simulink model "quad_12_1_r2021a"  (R2022a)
settings: Solver=ode4  StartTime=0.0  StopTime=120  FixedStep=0.001  RelTol=1e-3
values from neighbouring files (symbols this model uses):
  Ixc = 9373.661914436/1e6    (= 0.00937366191444)    [ParamsInit_test.m]
  Iyc = 11755.067703159/1e6    (= 0.0117550677032)    [ParamsInit_test.m]
  Izc = 17533.553367555/1e6    (= 0.0175335533676)    [ParamsInit_test.m]
  kd_h = damp_ratio_h*2*sqrt(kp_h*Vehicle.Airframe.mass)    [ParamsInit_test.m]
  kd_phi = damp_ratio_phi*2*sqrt(kp_phi*Ixc)    [ParamsInit_test.m]
  kd_theta = damp_ratio_theta*2*sqrt(kp_theta*Iyc)    [ParamsInit_test.m]
  kd_yaw = damp_ratio_yaw*2*sqrt(kp_yaw*Izc)    [ParamsInit_test.m]
  kp_h = omega_n_h^2*Vehicle.Airframe.mass    [ParamsInit_test.m]
  kp_phi = omega_n_phi^2*Ixc    (= 0.937366191444)    [ParamsInit_test.m]
  kp_position = 0.1    [ParamsInit_test.m]
  kp_theta = omega_n_theta^2*Iyc    (= 1.17550677032)    [ParamsInit_test.m]
  kp_vx = 0.25    [ParamsInit_test.m]
  kp_vy = 0.25    [ParamsInit_test.m]
  kp_yaw = omega_n_yaw^2*Izc    (= 0.0175335533676)    [ParamsInit_test.m]
undefined symbols (not defined in the file or in its folder): Vehicle
libraries: simulink x3, aerolibnav x3, aerolibconvert2 x2, mspfiltlib x1, sensorgpslib x1, mspsensorlib x1, sensorinslib x1, aerolibasang x1, sharedtransform x1, aerolibanimutils x1, uavutilslib x1
settings Model: Creator=gaowe  LastModifiedBy=GMS
settings SolverCC: AlgebraicLoopSolver=TrustRegion
settings RTWCC: DLArmComputeVersion=19.05

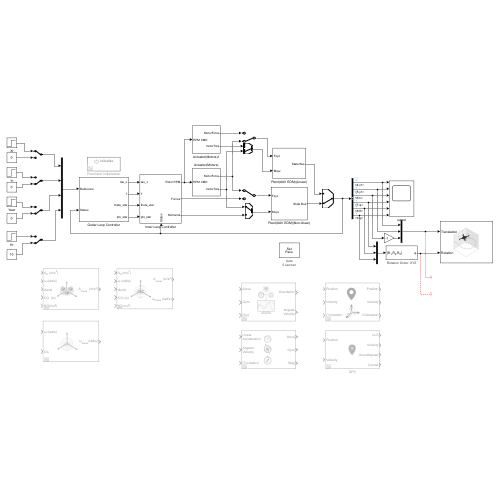
[thumbnail: Simulink's stored preview of the top-level diagram]
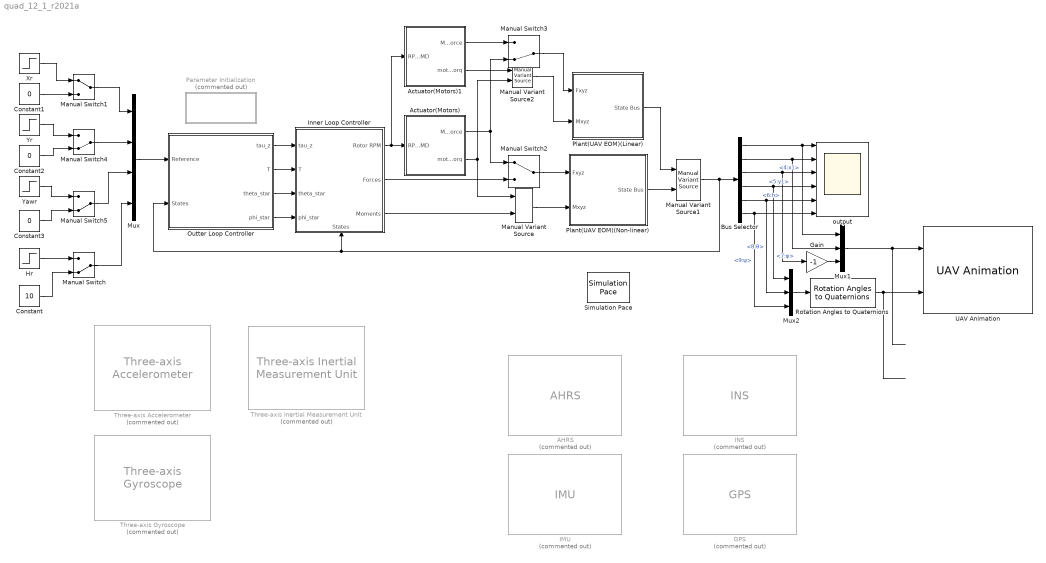
== system quad_12_1_r2021a ==
  AHRS : mspfiltlib/AHRS  Commented=on  DispRefFrame=NED  DecimationFactor=1  InitialProcessNoise=ahrsfilter.defaultProcessNoise  OrientationFormat=quaternion  SimulateUsing=Interpreted execution  AccelerometerNoise=0.0001924722  GyroscopeNoise=9.1385e-5  MagnetometerNoise=0.1  GyroscopeDriftNoise=3.0462e-13  LinearAccelerationNoise=0.0096236100000000012  MagneticDisturbanceNoise=0.5  LinearAccelerationDecayFactor=0.5  MagneticDisturbanceDecayFactor=0.5  ExpectedMagneticFieldStrength=50
  Actuator(Motors) : Subsystem
  Actuator(Motors)1 : Subsystem
  Bus Selector : BusSelector  OutputSignals=4:x1,5:y1,6:h,7:φ,8:θ,9:ψ
  Constant : Constant  Value=10
  Constant1 : Constant  Value=0
  Constant2 : Constant  Value=0
  Constant3 : Constant  Value=0
  GPS : sensorgpslib/GPS  Commented=on  DispRefFrame=NED  PositionInputFormat=Local  ReferenceLocation=[ 0, 0, 0 ]  HorizontalPositionAccuracy=1.6  VerticalPositionAccuracy=3  VelocityAccuracy=0.1  DecayFactor=0.999  SeedDouble=67  SimulateUsing=Interpreted execution
  Gain : Gain  Gain=-1
  Hr : Step  Time=0  After=20  SampleTime=0
  IMU : mspsensorlib/IMU  Commented=on  DispRefFrame=NED  Temperature=25  MagneticFieldNED=[ 27.5550, -2.4169, -16.0849 ]  MagneticFieldENU=[ -2.4169, 27.5550, 16.0849 ]  SeedDouble=67  SimulateUsing=Interpreted execution  AccelParamsMeasurementRange=Inf  AccelParamsResolution=0  AccelParamsConstantBias=[ 0, 0, 0 ]  AccelParamsAxesMisalignment=[ 100, 0, 0; 0, 100, 0; 0, 0, 100 ]  AccelParamsNoiseDensity=[ 0, 0, 0 ]  AccelParamsBiasInstability=[ 0, 0, 0 ]  AccelParamsRandomWalk=[ 0, 0, 0 ]  AccelParamsTemperatureBias=[ 0, 0, 0 ]  AccelParamsTemperatureScaleFactor=[ 0, 0, 0 ]  GyroParamsMeasurementRange=Inf  GyroParamsResolution=0  GyroParamsConstantBias=[ 0, 0, 0 ]  GyroParamsAxesMisalignment=[ 100, 0, 0; 0, 100, 0; 0, 0, 100 ]  GyroParamsAccelerationBias=[ 0, 0, 0 ]  GyroParamsNoiseDensity=[ 0, 0, 0 ]  GyroParamsBiasInstability=[ 0, 0, 0 ]  GyroParamsRandomWalk=[ 0, 0, 0 ]  GyroParamsTemperatureBias=[ 0, 0, 0 ]  GyroParamsTemperatureScaleFactor=[ 0, 0, 0 ]  MagParamsMeasurementRange=Inf  MagParamsResolution=0  MagParamsConstantBias=[ 0, 0, 0 ]  MagParamsAxesMisalignment=[ 100, 0, 0; 0, 100, 0; 0, 0, 100 ]  MagParamsNoiseDensity=[ 0, 0, 0 ]  MagParamsBiasInstability=[ 0, 0, 0 ]  MagParamsRandomWalk=[ 0, 0, 0 ]  MagParamsTemperatureBias=[ 0, 0, 0 ]  MagParamsTemperatureScaleFactor=[ 0, 0, 0 ]
  INS : sensorinslib/INS  Commented=on  MountingLocation=[0 0 0]  RollAccuracy=0.2  PitchAccuracy=0.2  YawAccuracy=1  PositionAccuracy=1  VelocityAccuracy=0.05  UseAccelAndAngVel=off  AccelerationAccuracy=0  AngularVelocityAccuracy=0  TimeInput=off  PositionErrorFactor=[0 0 0]  SeedDouble=67  SimulateUsing=Interpreted execution
  Inner Loop Controller : Subsystem
      settings: PortSchema="{\"entries\":[{\"content\":{\"sides\":[{\"content\":{\"connectorIds\":[\"In1\",\"In2\",\"In3\",\"In4\"]},\"type\":\"ConnectorPlacement.EquallySpacedRectSide\",\"uuid\":\"3024e14a-e42b-4ece-95b6-8188e577f7ea\"},{\"content\":{\"connectorIds\":[\"Out1\",\"Out2\",\"Out3\"],\"side\":\"RIGHT\"},\"type\":\"ConnectorPlacement.EquallySpacedRectSide\",\"uuid\":\"28791f10-00d9-435c-9b3a-62150bd300bc\"},{\"content\":{\"connectorIds\":[],\"side\":\"TOP\"},\"type\":\"ConnectorPlacement.EquallySpacedRectSide\",\"uuid\":\"5a81466d-668a-47df-a46c-2854fa138474\"},{\"content\":{\"connectorIds\":[\"In5\"],\"side\":\"BOTTOM\"},\"type\":\"ConnectorPlacement.EquallySpacedRectSide\",\"uuid\":\"dc01fcce-ea7b-43d7-98f8-2115160ba315\"}]},\"type\":\"ConnectorPlacement.EquallySpacedConnector\",\"uuid\":\"802a1a82-5ed7-4d3a-8fbf-5749d0aa0952\"}],\"packageUris\":[\"http://schema.mathworks.com/mf0/Connector/R2020b\"],\"version\":\"1.0\"}"
  Manual Variant Source : simulink/Signal Routing/Manual Variant Source  NumChoices=2  LabelModeActiveChoice=V_1
  Manual Variant Source1 : simulink/Signal Routing/Manual Variant Source  NumChoices=2  LabelModeActiveChoice=V_2
  Manual Variant Source2 : simulink/Signal Routing/Manual Variant Source  NumChoices=2  LabelModeActiveChoice=V_2
  Manual Switch{,3..5} (4 alike) : ManualSwitch  CurrentSetting=0
  Manual Switch1 : ManualSwitch
  Manual Switch2 : ManualSwitch
  Mux : Mux
  Mux1 : Mux  Inputs=3
  Mux2 : Mux  Inputs=3
  Outter Loop Controller : Subsystem
  Parameter Initialization : Subsystem  Commented=on  TreatAsAtomicUnit=on
  Plant(UAV EOM)(Linear) : Subsystem
  Plant(UAV EOM)(Non-linear) : Subsystem
  Rotation Angles to Quaternions : sharedtransform/Rotation Angles to Quaternions  rotationOrder=XYZ  aMode=aMode
  Simulation Pace : aerolibanimutils/Simulation Pace  SimulationPace=5  SleepMode=Auto  OutputPaceError=off  SampleTime=1/100
  Three-axis Accelerometer : aerolibnav/Three-axis Accelerometer  Commented=on  units=Metric (MKS)  acc=[0 0 0]  gtype=on  dtype_a=on  w_a=190  z_a=0.707  a_sf_cc=[1 0 0; 0 1 0; 0 0 1]  a_bias=[0 0 0]  a_Ts=0  a_rand=on  a_seeds=[23093 23094 23095]  a_pow=[0.001 0.001 0.001]  a_sat="[-inf  -inf  -inf  inf inf inf]"
  Three-axis Gyroscope : aerolibnav/Three-axis Gyroscope  Commented=on  dtype_g=on  w_g=190  z_g=0.707  g_sf_cc=[1 0 0; 0 1 0; 0 0 1]  g_bias=[0 0 0]  g_sen=[0 0 0]  g_Ts=0  g_rand=on  g_seeds=[23093 23094 23095]  g_pow=[0.0001 0.0001 0.0001]  g_sat="[-inf  -inf  -inf  inf inf inf]"
  Three-axis Inertial Measurement Unit : aerolibnav/Three-axis Inertial Measurement Unit  Commented=on  units=Metric (MKS)  imu=[0 0 0]  i_Ts=0  dtype_a=on  w_a=190  z_a=0.707  a_sf_cc=[1 0 0; 0 1 0; 0 0 1]  a_bias=[0 0 0]  a_sat="[-inf  -inf  -inf  inf inf inf]"  dtype_g=on  w_g=190  z_g=0.707  g_sf_cc=[1 0 0; 0 1 0; 0 0 1]  g_bias=[0 0 0]  g_sens=[0 0 0]  g_sat="[-inf  -inf  -inf  inf inf inf]"  i_rand=on  i_seeds=[23093 23094 23095 23096 23097 23098]  i_pow=[0.001 0.001 0.001 0.0001 0.0001 0.0001]
  UAV Animation : uavutilslib/UAV Animation  UAVType=Multirotor  UAVSize=1  InertialZDirection=Down  SampleTime=1/100
  Xr : Step  Time=0  After=10  SampleTime=0
  Yawr : Step  Time=0  After=pi/2  SampleTime=0
  Yr : Step  Time=0  After=10  SampleTime=0
  output : Scope  NumInputPorts=6
  wires:
  Manual Variant Source1/1 -> Outter Loop Controller/2(States), Inner Loop Controller/5(States), Bus Selector/1
  Mux/1 -> Outter Loop Controller/1(Reference)
  Manual Switch1/1 -> Mux/1
  Constant2/1 -> Manual Switch4/2
  Yawr/1 -> Manual Switch5/1
  Hr/1 -> Manual Switch/1
  Outter Loop Controller/3(theta_star) -> Inner Loop Controller/3(theta_star)
  Outter Loop Controller/1(tau_z) -> Inner Loop Controller/1(tau_z)
  Outter Loop Controller/2(T) -> Inner Loop Controller/2(T)
  Outter Loop Controller/4(phi_star) -> Inner Loop Controller/4(phi_star)
  Inner Loop Controller/1(Rotor RPM) -> Actuator(Motors)1/1(RPM CMD), Actuator(Motors)/1(RPM CMD)
  Actuator(Motors)/1(MotorForce) -> Manual Switch3/2, Manual Switch2/1
  Actuator(Motors)/2(motorTorq) -> Manual Variant Source2/2, Manual Variant Source/1
  Bus Selector/1 -> Mux1/1, output/1  "<4:x1>"
  Bus Selector/2 -> Mux1/2, output/2  "<5:y1>"
  Bus Selector/3 -> Gain/1, output/3  "<6:h>"
  Bus Selector/4 -> Mux2/1, output/4  "<7:φ>"
  Bus Selector/5 -> Mux2/2, output/5  "<8:θ>"
  Bus Selector/6 -> Mux2/3, output/6  "<9:ψ>"
  Manual Switch/1 -> Mux/4
  Constant/1 -> Manual Switch/2
  Constant1/1 -> Manual Switch1/2
  Xr/1 -> Manual Switch1/1
  Inner Loop Controller/2(Forces) -> Manual Switch2/2
  Inner Loop Controller/3(Moments) -> Manual Variant Source/2
  Plant(UAV EOM)(Linear)/1(State Bus) -> Manual Variant Source1/1
  Manual Variant Source/1 -> Plant(UAV EOM)(Non-linear)/2(Mxyz)
  Manual Switch2/1 -> Plant(UAV EOM)(Non-linear)/1(Fxyz)
  Plant(UAV EOM)(Non-linear)/1(State Bus) -> Manual Variant Source1/2
  Actuator(Motors)1/1(MotorForce) -> Manual Switch3/1
  Actuator(Motors)1/2(motorTorq) -> Manual Variant Source2/1
  Manual Switch3/1 -> Plant(UAV EOM)(Linear)/1(Fxyz)
  Manual Variant Source2/1 -> Plant(UAV EOM)(Linear)/2(Mxyz)
  Manual Switch4/1 -> Mux/2
  Yr/1 -> Manual Switch4/1
  Constant3/1 -> Manual Switch5/2
  Manual Switch5/1 -> Mux/3
  Mux1/1 -> UAV Animation/1
  Rotation Angles to Quaternions/1 -> UAV Animation/2
  Mux2/1 -> Rotation Angles to Quaternions/1
  Gain/1 -> Mux1/3

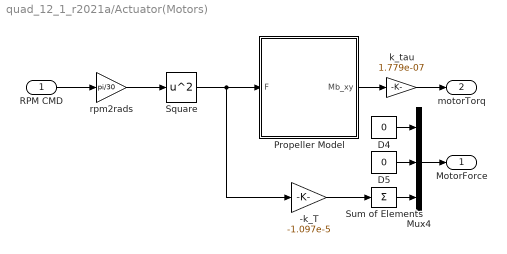
== system quad_12_1_r2021a/Actuator(Motors) ==
  RPM CMD : Inport
  -k_T : Gain  Gain=-1.097e-5
  D4 : Constant  Value=0
  D5 : Constant  Value=0
  Mux4 : Mux  Inputs=3
  Propeller Model : MATLAB Function  TreatAsAtomicUnit=on
  Square : Math  Operator=square
  Sum of Elements : Sum  Inputs=+
  k_tau : Gain  Gain=1.779e-07
  rpm2rads : Gain  Gain=pi/30
  MotorForce : Outport
  motorTorq : Outport  Port=2
  wires:
  k_tau/1 -> motorTorq/1
  Mux4/1 -> MotorForce/1
  Sum of Elements/1 -> Mux4/3
  -k_T/1 -> Sum of Elements/1
  Square/1 -> -k_T/1, Propeller Model/1(F)
  Propeller Model/1(Mb_xy) -> k_tau/1
  D4/1 -> Mux4/1
  D5/1 -> Mux4/2
  RPM CMD/1 -> rpm2rads/1
  rpm2rads/1 -> Square/1

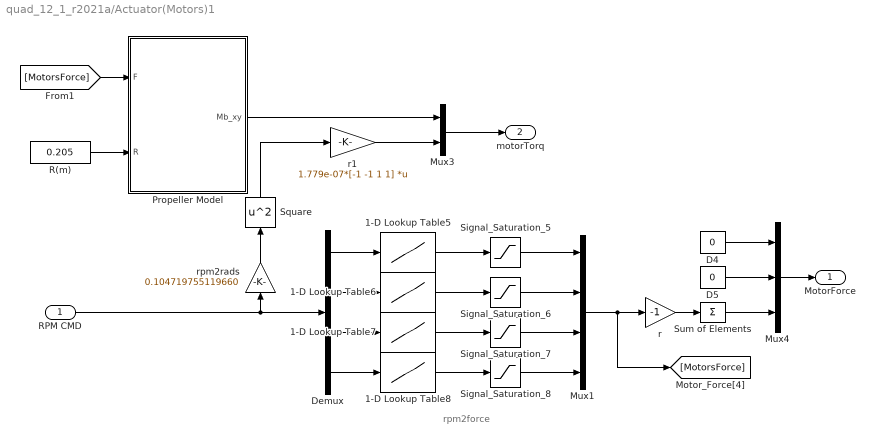
== system quad_12_1_r2021a/Actuator(Motors)1 ==
  note: rpm2force
  RPM CMD : Inport
  1-D Lookup Table5 : Lookup_n-D  NumberOfTableDimensions=1  BreakpointsForDimension1=|  BeginIndexSearchUsingPreviousIndexResult=on  Table=|  InternalRulePriority=Speed  RndMeth=Simplest
      BreakpointsForDimension1=|
      | [2847
      | 3689
      | 4585
      | 5400
      | 6400
      | 7000
      | 7800
      | 8222
      | 9300
      | 10700]
      Table=|
      | [0.6664
      | 1.4308
      | 2.3422
      | 3.3418
      | 4.9098
      | 5.929
      | 7.399
      | 7.6244
      | 10.976
      | 13.72]
  1-D Lookup Table6 : Lookup_n-D  NumberOfTableDimensions=1  BreakpointsForDimension1=|  BeginIndexSearchUsingPreviousIndexResult=on  Table=|  InternalRulePriority=Speed  RndMeth=Simplest
      BreakpointsForDimension1=|
      | [2847
      | 3689
      | 4585
      | 5400
      | 6400
      | 7000
      | 7800
      | 8222
      | 9300
      | 10700]
      Table=|
      | [0.6664
      | 1.4308
      | 2.3422
      | 3.3418
      | 4.9098
      | 5.929
      | 7.399
      | 7.6244
      | 10.976
      | 13.72]
  1-D Lookup Table7 : Lookup_n-D  NumberOfTableDimensions=1  BreakpointsForDimension1=|  BeginIndexSearchUsingPreviousIndexResult=on  Table=|  InternalRulePriority=Speed  RndMeth=Simplest
      BreakpointsForDimension1=|
      | [2847
      | 3689
      | 4585
      | 5400
      | 6400
      | 7000
      | 7800
      | 8222
      | 9300
      | 10700]
      Table=|
      | [0.6664
      | 1.4308
      | 2.3422
      | 3.3418
      | 4.9098
      | 5.929
      | 7.399
      | 7.6244
      | 10.976
      | 13.72]
  1-D Lookup Table8 : Lookup_n-D  NumberOfTableDimensions=1  BreakpointsForDimension1=|  BeginIndexSearchUsingPreviousIndexResult=on  Table=|  InternalRulePriority=Speed  RndMeth=Simplest
      BreakpointsForDimension1=|
      | [2847
      | 3689
      | 4585
      | 5400
      | 6400
      | 7000
      | 7800
      | 8222
      | 9300
      | 10700]
      Table=|
      | [0.6664
      | 1.4308
      | 2.3422
      | 3.3418
      | 4.9098
      | 5.929
      | 7.399
      | 7.6244
      | 10.976
      | 13.72]
  D4 : Constant  Value=0
  D5 : Constant  Value=0
  Demux : Demux
  Mux1 : Mux
  Mux3 : Mux  Inputs=[2 1]
  Mux4 : Mux  Inputs=3
  Propeller Model : MATLAB Function  TreatAsAtomicUnit=on
  R(m) : Constant  Value=0.205
  Signal_Saturation_{5..8} (4 alike) : Saturate  UpperLimit=1.4*9.8  LowerLimit=0
  Square : Math  Operator=square
  Sum of Elements : Sum  Inputs=+
  r : Gain  Gain=-1
  r1 : Gain  Gain=1.779e-07*[-1 -1 1 1]  Multiplication=Matrix(K*u)
  rpm2rads : Gain  Gain=0.104719755119660
  MotorForce : Outport
  motorTorq : Outport  Port=2
  wires:
  Signal_Saturation_6/1 -> Mux1/2
  1-D Lookup Table7/1 -> Signal_Saturation_7/1
  Mux3/1 -> motorTorq/1
  1-D Lookup Table6/1 -> Signal_Saturation_6/1
  Mux4/1 -> MotorForce/1
  r1/1 -> Mux3/2
  Sum of Elements/1 -> Mux4/3
  r/1 -> Sum of Elements/1
  Mux1/1 -> [MotorsForce], r/1
  Demux/1 -> 1-D Lookup Table5/1
  Square/1 -> r1/1
  1-D Lookup Table5/1 -> Signal_Saturation_5/1
  Demux/3 -> 1-D Lookup Table7/1
  Signal_Saturation_5/1 -> Mux1/1
  1-D Lookup Table8/1 -> Signal_Saturation_8/1
  [MotorsForce] -> Propeller Model/1(F)
  Demux/4 -> 1-D Lookup Table8/1
  Demux/2 -> 1-D Lookup Table6/1
  Signal_Saturation_7/1 -> Mux1/3
  Propeller Model/1(Mb_xy) -> Mux3/1
  Signal_Saturation_8/1 -> Mux1/4
  R(m)/1 -> Propeller Model/2(R)
  D4/1 -> Mux4/1
  D5/1 -> Mux4/2
  RPM CMD/1 -> Demux/1, rpm2rads/1
  rpm2rads/1 -> Square/1

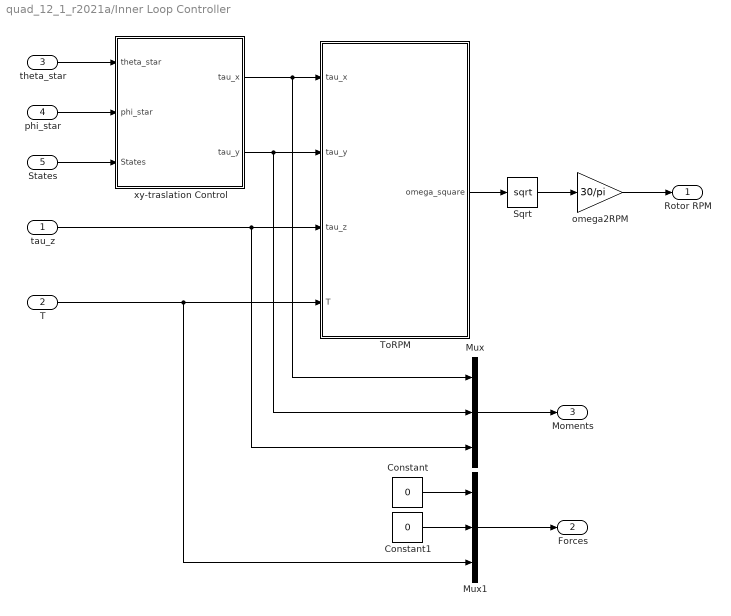
== system quad_12_1_r2021a/Inner Loop Controller ==
  tau_z : Inport
  T : Inport  Port=2
  theta_star : Inport  Port=3
  phi_star : Inport  Port=4
  States : Inport  Port=5
  Constant : Constant  Value=0
  Constant1 : Constant  Value=0
  Mux : Mux  Inputs=3
  Mux1 : Mux  Inputs=3
  Sqrt : Sqrt
  ToRPM : MATLAB Function  TreatAsAtomicUnit=on
  omega2RPM : Gain  Gain=30/pi
  xy-traslation Control : Subsystem
  Rotor RPM : Outport
  Forces : Outport  Port=2
  Moments : Outport  Port=3
  wires:
  theta_star/1 -> xy-traslation Control/1(theta_star)
  States/1 -> xy-traslation Control/3(States)
  phi_star/1 -> xy-traslation Control/2(phi_star)
  tau_z/1 -> Mux/3, ToRPM/3(tau_z)
  xy-traslation Control/2(tau_y) -> Mux/2, ToRPM/2(tau_y)
  xy-traslation Control/1(tau_x) -> Mux/1, ToRPM/1(tau_x)
  Sqrt/1 -> omega2RPM/1
  omega2RPM/1 -> Rotor RPM/1
  ToRPM/1(omega_square) -> Sqrt/1
  Mux/1 -> Moments/1
  Constant/1 -> Mux1/1
  Constant1/1 -> Mux1/2
  Mux1/1 -> Forces/1
  T/1 -> Mux1/3, ToRPM/4(T)

== system quad_12_1_r2021a/Outter Loop Controller ==
  Reference : Inport
  States : Inport  Port=2
  Demux : Demux
  Height Control : Subsystem
  Position Control : Subsystem
  Velocity Control : Subsystem
  Yaw Control : Subsystem
  tau_z : Outport
  T : Outport  Port=2
  theta_star : Outport  Port=3
  phi_star : Outport  Port=4
  wires:
  Reference/1 -> Demux/1
  States/1 -> Position Control/3(States), Velocity Control/3(States), Yaw Control/2(States), Height Control/2(States)
  Velocity Control/1(theta_star) -> theta_star/1
  Demux/4 -> Height Control/1(Hr)  "Hr"
  Demux/3 -> Yaw Control/1(Yawr)  "Yawr"
  Demux/2 -> Position Control/2(yr)  "Yr"
  Demux/1 -> Position Control/1(xr)  "Xr"
  Height Control/1(T) -> T/1
  Yaw Control/1(tau_z) -> tau_z/1
  Velocity Control/2(phi_star) -> phi_star/1
  Position Control/1(vxr) -> Velocity Control/1(vxr)
  Position Control/2(vyr) -> Velocity Control/2(vyr)

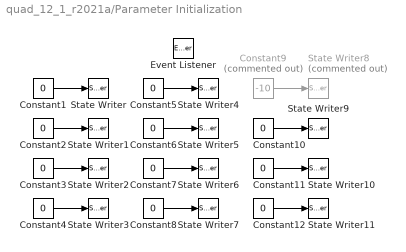
== system quad_12_1_r2021a/Parameter Initialization ==
  Constant{1..8,10..12} (11 alike) : Constant  Value=0
  Constant9 : Constant  Commented=on  Value=-10
  Event Listener : EventListener  DisableCoverage=on  EventName=reset
  State Writer : StateWriter  StateOwnerBlock=../../Plant(UAV EOM)(Non-linear)/6DOF CORE/Subsystem9/Xe0
  State Writer1 : StateWriter  StateOwnerBlock=../../Plant(UAV EOM)(Non-linear)/6DOF CORE/Subsystem10/U0
  State Writer10 : StateWriter  StateOwnerBlock=../../Plant(UAV EOM)(Non-linear)/6DOF CORE/Subsystem/R0
  State Writer11 : StateWriter  StateOwnerBlock=../../Plant(UAV EOM)(Non-linear)/6DOF CORE/Subsystem6/ψ0
  State Writer2 : StateWriter  StateOwnerBlock=../../Plant(UAV EOM)(Non-linear)/6DOF CORE/Subsystem/P0
  State Writer3 : StateWriter  StateOwnerBlock=../../Plant(UAV EOM)(Non-linear)/6DOF CORE/Subsystem6/θ0
  State Writer4 : StateWriter  StateOwnerBlock=../../Plant(UAV EOM)(Non-linear)/6DOF CORE/Subsystem9/Ye0
  State Writer5 : StateWriter  StateOwnerBlock=../../Plant(UAV EOM)(Non-linear)/6DOF CORE/Subsystem10/V0
  State Writer6 : StateWriter  StateOwnerBlock=../../Plant(UAV EOM)(Non-linear)/6DOF CORE/Subsystem/Q0
  State Writer7 : StateWriter  StateOwnerBlock=../../Plant(UAV EOM)(Non-linear)/6DOF CORE/Subsystem6/φ0
  State Writer8 : StateWriter  Commented=on  StateOwnerBlock=../../Plant(UAV EOM)(Non-linear)/6DOF CORE/Subsystem9/Ze0
  State Writer9 : StateWriter  StateOwnerBlock=../../Plant(UAV EOM)(Non-linear)/6DOF CORE/Subsystem10/W0
  wires:
  Constant1/1 -> State Writer/1
  Constant2/1 -> State Writer1/1
  Constant4/1 -> State Writer3/1
  Constant3/1 -> State Writer2/1
  Constant6/1 -> State Writer5/1
  Constant7/1 -> State Writer6/1
  Constant5/1 -> State Writer4/1
  Constant8/1 -> State Writer7/1
  Constant10/1 -> State Writer9/1
  Constant11/1 -> State Writer10/1
  Constant9/1 -> State Writer8/1
  Constant12/1 -> State Writer11/1

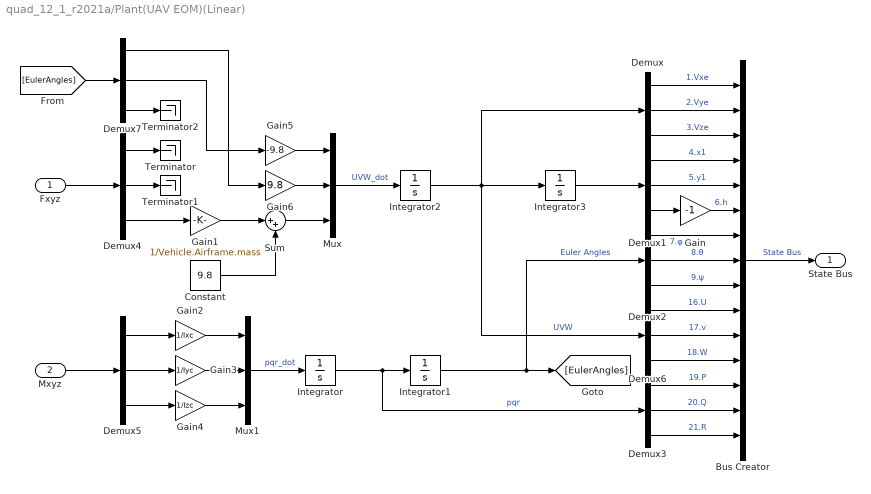
== system quad_12_1_r2021a/Plant(UAV EOM)(Linear) ==
  Fxyz : Inport
  Mxyz : Inport  Port=2
  Bus Creator : BusCreator  Inputs=15
  Constant : Constant  Value=9.8
  Demux{,1..7} (8 alike) : Demux  Outputs=3
  Gain : Gain  Gain=-1
  Gain1 : Gain  Gain=1/Vehicle.Airframe.mass
  Gain2 : Gain  Gain=1/Ixc
  Gain3 : Gain  Gain=1/Iyc
  Gain4 : Gain  Gain=1/Izc
  Gain5 : Gain  Gain=-9.8
  Gain6 : Gain  Gain=9.8
  Integrator : Integrator  InitialCondition=[0,0,0]
  Integrator1 : Integrator  InitialCondition=[0,0,0]
  Integrator2 : Integrator  InitialCondition=[0,0,0]
  Integrator3 : Integrator  InitialCondition=[0,0,-10]
  Mux : Mux  Inputs=3
  Mux1 : Mux  Inputs=3
  Sum : Sum  Inputs=|++
  Terminator : Terminator
  Terminator1 : Terminator
  Terminator2 : Terminator
  State Bus : Outport
  wires:
  Gain/1 -> Bus Creator/6  "6.h"
  Demux/1 -> Bus Creator/1  "1.Vxe"
  Demux6/2 -> Bus Creator/11  "17.v"
  Demux3/3 -> Bus Creator/15  "21.R"
  Demux3/1 -> Bus Creator/13  "19.P"
  Demux6/1 -> Bus Creator/10  "16.U"
  Demux2/2 -> Bus Creator/8  "8.θ"
  Demux2/1 -> Bus Creator/7  "7.φ"
  Demux1/3 -> Gain/1
  Demux2/3 -> Bus Creator/9  "9.ψ"
  Demux1/2 -> Bus Creator/5  "5.y1"
  Demux3/2 -> Bus Creator/14  "20.Q"
  Demux6/3 -> Bus Creator/12  "18.W"
  Demux/3 -> Bus Creator/3  "3.Vze"
  Demux1/1 -> Bus Creator/4  "4.x1"
  Demux/2 -> Bus Creator/2  "2.Vye"
  Bus Creator/1 -> State Bus/1  "State Bus"
  Fxyz/1 -> Demux4/1
  Mxyz/1 -> Demux5/1
  Demux4/1 -> Terminator/1
  Demux4/2 -> Terminator1/1
  Demux4/3 -> Gain1/1
  Gain1/1 -> Sum/1
  Demux5/2 -> Gain3/1
  Demux5/1 -> Gain2/1
  Demux5/3 -> Gain4/1
  Mux1/1 -> Integrator/1  "pqr_dot"
  Gain3/1 -> Mux1/2
  Gain2/1 -> Mux1/1
  Gain4/1 -> Mux1/3
  Integrator/1 -> Demux3/1, Integrator1/1  "pqr"
  Integrator1/1 -> [EulerAngles], Demux2/1  "Euler Angles"
  Gain5/1 -> Mux/1
  [EulerAngles] -> Demux7/1
  Demux7/1 -> Gain6/1
  Demux7/2 -> Gain5/1
  Gain6/1 -> Mux/2
  Demux7/3 -> Terminator2/1
  Mux/1 -> Integrator2/1  "UVW_dot"
  Integrator2/1 -> Demux/1, Integrator3/1, Demux6/1  "UVW"
  Integrator3/1 -> Demux1/1
  Constant/1 -> Sum/2
  Sum/1 -> Mux/3

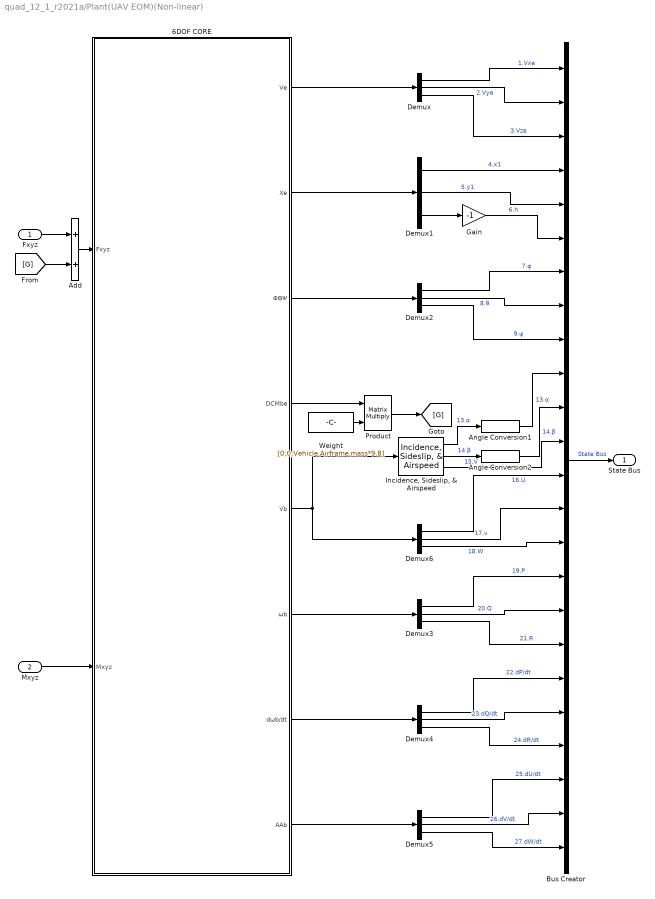
== system quad_12_1_r2021a/Plant(UAV EOM)(Non-linear) ==
  Fxyz : Inport
  Mxyz : Inport  Port=2
  6DOF CORE : Subsystem
  Add : Sum
  Angle Conversion1 : aerolibconvert2/Angle Conversion  IU=rad  OU=deg
  Angle Conversion2 : aerolibconvert2/Angle Conversion  IU=rad  OU=deg
  Bus Creator : BusCreator  Inputs=24
  Demux{,1..6} (7 alike) : Demux  Outputs=3
  Gain : Gain  Gain=-1
  "Incidence, Sideslip, & Airspeed" : aerolibasang/Incidence, Sideslip, & Airspeed
  Product : Product  Multiplication=Matrix(*)
  Weight : Constant  Value=[0;0;Vehicle.Airframe.mass*9.8]  VectorParams1D=off
  State Bus : Outport
  wires:
  Gain/1 -> Bus Creator/6  "6.h"
  6DOF CORE/5(Vb) -> "Incidence, Sideslip, & Airspeed"/1, Demux6/1
  6DOF CORE/1(Ve) -> Demux/1
  Demux/1 -> Bus Creator/1  "1.Vxe"
  Demux6/2 -> Bus Creator/14  "17.v"
  6DOF CORE/3(ΦΘΨ) -> Demux2/1
  Demux3/3 -> Bus Creator/18  "21.R"
  Demux5/3 -> Bus Creator/24  "27.dW/dt"
  Demux4/3 -> Bus Creator/21  "24.dR/dt"
  "Incidence, Sideslip, & Airspeed"/3 -> Bus Creator/12  "15.V"
  Demux3/1 -> Bus Creator/16  "19.P"
  Demux6/1 -> Bus Creator/13  "16.U"
  6DOF CORE/7(dωb/dt) -> Demux4/1
  Demux2/2 -> Bus Creator/8  "8.θ"
  Demux2/1 -> Bus Creator/7  "7.φ"
  "Incidence, Sideslip, & Airspeed"/1 -> Angle Conversion1/1  "13.α"
  6DOF CORE/6(ωb) -> Demux3/1
  Demux1/3 -> Gain/1
  6DOF CORE/2(Xe) -> Demux1/1
  Demux2/3 -> Bus Creator/9  "9.ψ"
  Demux4/2 -> Bus Creator/20  "23.dQ/dt"
  Demux5/2 -> Bus Creator/23  "26.dV/dt"
  Demux1/2 -> Bus Creator/5  "5.y1"
  Demux3/2 -> Bus Creator/17  "20.Q"
  Angle Conversion2/1 -> Bus Creator/11  "14.β"
  Demux5/1 -> Bus Creator/22  "25.dU/dt"
  Demux6/3 -> Bus Creator/15  "18.W"
  6DOF CORE/8(AAb) -> Demux5/1
  Demux4/1 -> Bus Creator/19  "22.dP/dt"
  Angle Conversion1/1 -> Bus Creator/10  "13.α"
  Demux/3 -> Bus Creator/3  "3.Vze"
  "Incidence, Sideslip, & Airspeed"/2 -> Angle Conversion2/1  "14.β"
  Demux1/1 -> Bus Creator/4  "4.x1"
  Demux/2 -> Bus Creator/2  "2.Vye"
  Bus Creator/1 -> State Bus/1  "State Bus"
  Fxyz/1 -> Add/1
  Mxyz/1 -> 6DOF CORE/2(Mxyz)
  Product/1 -> [G]
  Weight/1 -> Product/2
  6DOF CORE/4(DCMbe) -> Product/1
  [G] -> Add/2
  Add/1 -> 6DOF CORE/1(Fxyz)

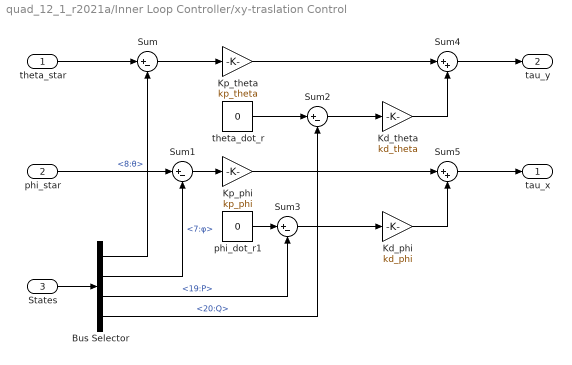
== system quad_12_1_r2021a/Inner Loop Controller/xy-traslation Control ==
  theta_star : Inport
  phi_star : Inport  Port=2
  States : Inport  Port=3
  Bus Selector : BusSelector  OutputSignals=8:θ,7:φ,19:P,20:Q
  Kd_phi : Gain  Gain=kd_phi
  Kd_theta : Gain  Gain=kd_theta
  Kp_phi : Gain  Gain=kp_phi
  Kp_theta : Gain  Gain=kp_theta
  Sum{,1..3} (4 alike) : Sum  Inputs=|+-
  Sum4 : Sum  Inputs=|++
  Sum5 : Sum  Inputs=|++
  phi_dot_r1 : Constant  Value=0
  theta_dot_r : Constant  Value=0
  tau_x : Outport
  tau_y : Outport  Port=2
  wires:
  theta_star/1 -> Sum/1
  States/1 -> Bus Selector/1
  Bus Selector/1 -> Sum/2  "<8:θ>"
  phi_star/1 -> Sum1/1
  Bus Selector/2 -> Sum1/2  "<7:φ>"
  Sum/1 -> Kp_theta/1
  Sum1/1 -> Kp_phi/1
  Bus Selector/3 -> Sum3/2  "<19:P>"
  Bus Selector/4 -> Sum2/2  "<20:Q>"
  Kp_theta/1 -> Sum4/1
  theta_dot_r/1 -> Sum2/1
  Kp_phi/1 -> Sum5/1
  Sum2/1 -> Kd_theta/1
  Kd_theta/1 -> Sum4/2
  Sum4/1 -> tau_y/1
  phi_dot_r1/1 -> Sum3/1
  Sum3/1 -> Kd_phi/1
  Sum5/1 -> tau_x/1
  Kd_phi/1 -> Sum5/2

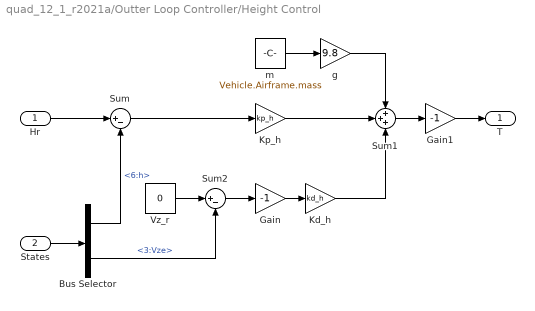
== system quad_12_1_r2021a/Outter Loop Controller/Height Control ==
  Hr : Inport
  States : Inport  Port=2
  Bus Selector : BusSelector  OutputSignals=6:h,3:Vze
  Gain : Gain  Gain=-1
  Gain1 : Gain  Gain=-1
  Kd_h : Gain  Gain=kd_h
  Kp_h : Gain  Gain=kp_h
  Sum : Sum  Inputs=|+-
  Sum1 : Sum  Inputs=+++
  Sum2 : Sum  Inputs=|+-
  Vz_r : Constant  Value=0
  g : Gain  Gain=9.8
  m : Constant  Value=Vehicle.Airframe.mass
  T : Outport
  wires:
  Sum1/1 -> Gain1/1
  States/1 -> Bus Selector/1
  Hr/1 -> Sum/1
  Bus Selector/1 -> Sum/2  "<6:h>"
  Sum/1 -> Kp_h/1
  Kd_h/1 -> Sum1/3
  Bus Selector/2 -> Sum2/2  "<3:Vze>"
  m/1 -> g/1
  g/1 -> Sum1/1
  Sum2/1 -> Gain/1
  Kp_h/1 -> Sum1/2
  Gain/1 -> Kd_h/1
  Gain1/1 -> T/1
  Vz_r/1 -> Sum2/1

== system quad_12_1_r2021a/Outter Loop Controller/Position Control ==
  xr : Inport
  yr : Inport  Port=2
  States : Inport  Port=3
  Bus Selector : BusSelector  OutputSignals=4:x1,5:y1,9:ψ
  Kp_position : Gain  Gain=kp_position
  MATLAB Function : MATLAB Function  TreatAsAtomicUnit=on
  Mux : Mux  Inputs=2
  Sum : Sum  Inputs=|+-
  Sum1 : Sum  Inputs=|+-
  vxr : Outport
  vyr : Outport  Port=2
  wires:
  xr/1 -> Sum/1
  MATLAB Function/1(vxr) -> vxr/1  "vxr"
  MATLAB Function/2(vyr) -> vyr/1  "vyr"
  States/1 -> Bus Selector/1
  Bus Selector/3 -> MATLAB Function/2(psi)  "<9:ψ>"
  Bus Selector/2 -> Sum1/2  "<5:y1>"
  Bus Selector/1 -> Sum/2  "<4:x1>"
  yr/1 -> Sum1/1
  Mux/1 -> Kp_position/1
  Sum1/1 -> Mux/2
  Kp_position/1 -> MATLAB Function/1(v)
  Sum/1 -> Mux/1

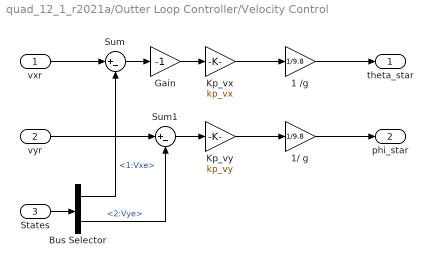
== system quad_12_1_r2021a/Outter Loop Controller/Velocity Control ==
  vxr : Inport
  vyr : Inport  Port=2
  States : Inport  Port=3
  1 /g : Gain  Gain=1/9.8
  1/ g : Gain  Gain=1/9.8
  Bus Selector : BusSelector  OutputSignals=1:Vxe,2:Vye
  Gain : Gain  Gain=-1
  Kp_vx : Gain  Gain=kp_vx
  Kp_vy : Gain  Gain=kp_vy
  Sum : Sum  Inputs=|+-
  Sum1 : Sum  Inputs=|+-
  theta_star : Outport
  phi_star : Outport  Port=2
  wires:
  vxr/1 -> Sum/1
  vyr/1 -> Sum1/1
  Sum/1 -> Gain/1
  1 /g/1 -> theta_star/1
  1/ g/1 -> phi_star/1
  Kp_vx/1 -> 1 /g/1
  Sum1/1 -> Kp_vy/1
  Kp_vy/1 -> 1/ g/1
  States/1 -> Bus Selector/1
  Bus Selector/1 -> Sum/2  "<1:Vxe>"
  Bus Selector/2 -> Sum1/2  "<2:Vye>"
  Gain/1 -> Kp_vx/1

== system quad_12_1_r2021a/Outter Loop Controller/Yaw Control ==
  Yawr : Inport
  States : Inport  Port=2
  Bus Selector : BusSelector  OutputSignals=9:ψ,21:R
  Kd_yaw : Gain  Gain=kd_yaw
  Kp_yaw : Gain  Gain=kp_yaw
  Sum : Sum  Inputs=|+-
  Sum1 : Sum  Inputs=|+-
  Sum2 : Sum  Inputs=|++
  Yaw_dot_r : Constant  Value=0
  tau_z : Outport
  wires:
  Sum2/1 -> tau_z/1
  Yawr/1 -> Sum/1
  Bus Selector/1 -> Sum/2  "<9:ψ>"
  Sum/1 -> Kp_yaw/1
  States/1 -> Bus Selector/1
  Bus Selector/2 -> Sum1/2  "<21:R>"
  Yaw_dot_r/1 -> Sum1/1
  Sum1/1 -> Kd_yaw/1
  Kp_yaw/1 -> Sum2/1
  Kd_yaw/1 -> Sum2/2

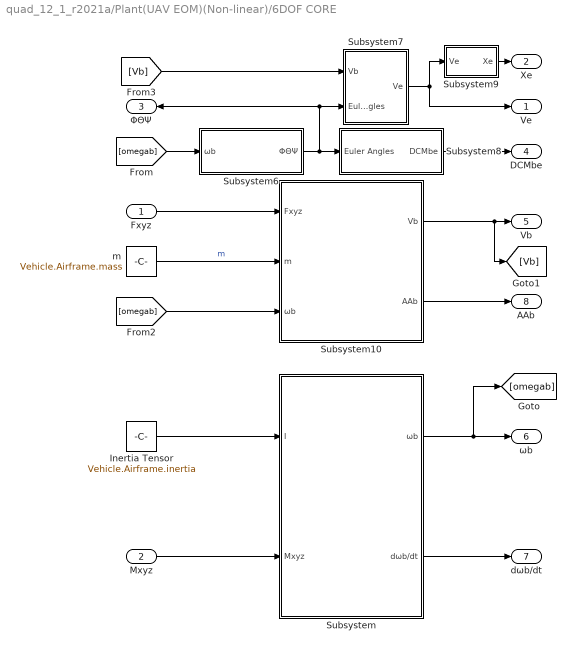
== system quad_12_1_r2021a/Plant(UAV EOM)(Non-linear)/6DOF CORE ==
  Fxyz : Inport
  Mxyz : Inport  Port=2
  Inertia Tensor : Constant  Value=Vehicle.Airframe.inertia  VectorParams1D=off
  Subsystem : Subsystem
  Subsystem10 : Subsystem
  Subsystem6 : Subsystem
  Subsystem7 : Subsystem
      settings: PortSchema="{\"entries\":[{\"content\":{\"sides\":[{\"content\":{\"connectorIds\":[]},\"type\":\"ConnectorPlacement.EquallySpacedRectSide\",\"uuid\":\"1bd4c84a-8e3a-484f-b157-4fc2072173e9\"},{\"content\":{\"connectorIds\":[],\"side\":\"RIGHT\"},\"type\":\"ConnectorPlacement.EquallySpacedRectSide\",\"uuid\":\"5d02806b-ecd1-4a3d-b653-3060473a0baf\"},{\"content\":{\"connectorIds\":[\"Out1\"],\"side\":\"TOP\"},\"type\":\"ConnectorPlacement.EquallySpacedRectSide\",\"uuid\":\"b006a162-3e36-45b5-99bc-3480dd68e666\"},{\"content\":{\"connectorIds\":[\"In1\",\"In2\"],\"side\":\"BOTTOM\"},\"type\":\"ConnectorPlacement.EquallySpacedRectSide\",\"uuid\":\"a3921935-1893-4001-94f5-fd44c1c6a502\"},{\"content\":{\"connectorIds\":[],\"side\":\"HIDDEN\"},\"type\":\"ConnectorPlacement.EquallySpacedRectSide\",\"uuid\":\"8e011310-df3e-4a51-a6dd-e16af6e4adf7\"}]},\"type\":\"ConnectorPlacement.EquallySpacedConnector\",\"uuid\":\"87633363-c957-4eb9-bec4-3afb23cb2e66\"}],\"packageUris\":[\"http://schema.mathworks.com/mf0/Connector/R2020b\"],\"version\":\"1.0\"}"
  Subsystem8 : Subsystem
  Subsystem9 : Subsystem
  m : Constant  Value=Vehicle.Airframe.mass
  Ve : Outport
  Xe : Outport  Port=2
  ΦΘΨ : Outport  Port=3
  DCMbe : Outport  Port=4
  Vb : Outport  Port=5
  ωb : Outport  Port=6
  dωb/dt : Outport  Port=7
  AAb : Outport  Port=8
  wires:
  Subsystem9/1(Xe) -> Xe/1
  Subsystem8/1(DCMbe) -> DCMbe/1
  Subsystem7/1(Ve) -> Subsystem9/1(Ve), Ve/1
  Subsystem6/1(ΦΘΨ) -> Subsystem7/2(Euler Angles), ΦΘΨ/1, Subsystem8/1(Euler Angles)
  [omegab] -> Subsystem6/1(ωb)
  [Vb] -> Subsystem7/1(Vb)
  Subsystem10/1(Vb) -> [Vb], Vb/1
  Fxyz/1 -> Subsystem10/1(Fxyz)
  m/1 -> Subsystem10/2(m)  "m"
  [omegab] -> Subsystem10/3(ωb)
  Subsystem10/2(AAb) -> AAb/1
  Subsystem/1(ωb) -> [omegab], ωb/1
  Mxyz/1 -> Subsystem/2(Mxyz)
  Subsystem/2(dωb/dt) -> dωb/dt/1
  Inertia Tensor/1 -> Subsystem/1(I)

== system quad_12_1_r2021a/Plant(UAV EOM)(Non-linear)/6DOF CORE/Subsystem ==
  I : Inport
  Mxyz : Inport  Port=2
  MATLAB Function : MATLAB Function  TreatAsAtomicUnit=on
  Mux4 : Mux  Inputs=3
  Mux5 : Mux  Inputs=3
  P0 : Integrator
  Q0 : Integrator
  R0 : Integrator
  ωb : Outport
  dωb/dt : Outport  Port=2
  wires:
  Q0/1 -> Mux4/2  "Q"
  MATLAB Function/2(Q_dot) -> Mux5/2, Q0/1  "dQ/dt"
  P0/1 -> Mux4/1  "P"
  MATLAB Function/1(P_dot) -> Mux5/1, P0/1  "dP/dt"
  MATLAB Function/3(R_dot) -> Mux5/3, R0/1  "dR/dt"
  R0/1 -> Mux4/3  "R"
  Mux5/1 -> dωb/dt/1
  Mxyz/1 -> MATLAB Function/2(M)
  I/1 -> MATLAB Function/1(I)
  Mux4/1 -> MATLAB Function/3(omega), ωb/1

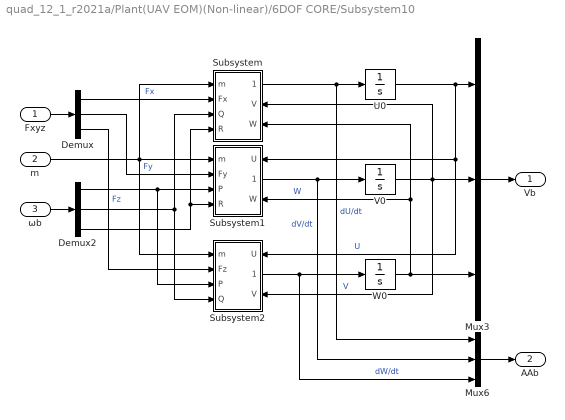
== system quad_12_1_r2021a/Plant(UAV EOM)(Non-linear)/6DOF CORE/Subsystem10 ==
  Fxyz : Inport
  m : Inport  Port=2
  ωb : Inport  Port=3
  Demux : Demux  Outputs=3
  Demux2 : Demux  Outputs=3
  Mux3 : Mux  Inputs=3
  Mux6 : Mux  Inputs=3
  Subsystem : Subsystem
      settings: PortSchema="{\"entries\":[{\"content\":{\"sides\":[{\"content\":{\"connectorIds\":[\"In1\",\"In2\",\"In3\",\"In4\"]},\"type\":\"ConnectorPlacement.EquallySpacedRectSide\",\"uuid\":\"326daed8-e070-42c4-b922-a1cfd1075610\"},{\"content\":{\"connectorIds\":[\"Out1\",\"In5\",\"In6\"],\"side\":\"RIGHT\"},\"type\":\"ConnectorPlacement.EquallySpacedRectSide\",\"uuid\":\"accd66e9-544e-4c99-a98b-e3a864bc5f81\"},{\"content\":{\"connectorIds\":[],\"side\":\"TOP\"},\"type\":\"ConnectorPlacement.EquallySpacedRectSide\",\"uuid\":\"83c3f4fc-532b-43a1-b874-56a52f4ca207\"},{\"content\":{\"connectorIds\":[],\"side\":\"HIDDEN\"},\"type\":\"ConnectorPlacement.EquallySpacedRectSide\",\"uuid\":\"414a66aa-d5b6-4143-97b4-f1301075a4c5\"}]},\"type\":\"ConnectorPlacement.EquallySpacedConnector\",\"uuid\":\"8a44064a-2e10-45f9-b0ec-d6ec6baf7018\"}],\"packageUris\":[\"http://schema.mathworks.com/mf0/Connector/R2020b\"],\"version\":\"1.0\"}"
  Subsystem1 : Subsystem
      settings: PortSchema="{\"entries\":[{\"content\":{\"sides\":[{\"content\":{\"connectorIds\":[\"In1\",\"In2\",\"In3\",\"In4\"]},\"type\":\"ConnectorPlacement.EquallySpacedRectSide\",\"uuid\":\"326daed8-e070-42c4-b922-a1cfd1075610\"},{\"content\":{\"connectorIds\":[\"In5\",\"Out1\",\"In6\"],\"side\":\"RIGHT\"},\"type\":\"ConnectorPlacement.EquallySpacedRectSide\",\"uuid\":\"accd66e9-544e-4c99-a98b-e3a864bc5f81\"},{\"content\":{\"connectorIds\":[],\"side\":\"TOP\"},\"type\":\"ConnectorPlacement.EquallySpacedRectSide\",\"uuid\":\"83c3f4fc-532b-43a1-b874-56a52f4ca207\"},{\"content\":{\"connectorIds\":[],\"side\":\"HIDDEN\"},\"type\":\"ConnectorPlacement.EquallySpacedRectSide\",\"uuid\":\"414a66aa-d5b6-4143-97b4-f1301075a4c5\"}]},\"type\":\"ConnectorPlacement.EquallySpacedConnector\",\"uuid\":\"8a44064a-2e10-45f9-b0ec-d6ec6baf7018\"}],\"packageUris\":[\"http://schema.mathworks.com/mf0/Connector/R2020b\"],\"version\":\"1.0\"}"
  Subsystem2 : Subsystem
      settings: PortSchema="{\"entries\":[{\"content\":{\"sides\":[{\"content\":{\"connectorIds\":[\"In1\",\"In2\",\"In3\",\"In4\"]},\"type\":\"ConnectorPlacement.EquallySpacedRectSide\",\"uuid\":\"326daed8-e070-42c4-b922-a1cfd1075610\"},{\"content\":{\"connectorIds\":[\"In5\",\"Out1\",\"In6\"],\"side\":\"RIGHT\"},\"type\":\"ConnectorPlacement.EquallySpacedRectSide\",\"uuid\":\"accd66e9-544e-4c99-a98b-e3a864bc5f81\"},{\"content\":{\"connectorIds\":[],\"side\":\"TOP\"},\"type\":\"ConnectorPlacement.EquallySpacedRectSide\",\"uuid\":\"83c3f4fc-532b-43a1-b874-56a52f4ca207\"},{\"content\":{\"connectorIds\":[],\"side\":\"HIDDEN\"},\"type\":\"ConnectorPlacement.EquallySpacedRectSide\",\"uuid\":\"414a66aa-d5b6-4143-97b4-f1301075a4c5\"}]},\"type\":\"ConnectorPlacement.EquallySpacedConnector\",\"uuid\":\"8a44064a-2e10-45f9-b0ec-d6ec6baf7018\"}],\"packageUris\":[\"http://schema.mathworks.com/mf0/Connector/R2020b\"],\"version\":\"1.0\"}"
  U0 : Integrator
  V0 : Integrator
  W0 : Integrator
  Vb : Outport
  AAb : Outport  Port=2
  wires:
  Subsystem2/1(dW/dt) -> Mux6/3, W0/1  "dW/dt"
  Demux2/3 -> Subsystem/4(R), Subsystem1/4(R)
  Demux/3 -> Subsystem2/2(Fz)  "Fz"
  V0/1 -> Mux3/2, Subsystem/5(V), Subsystem2/6(V)  "V"
  Subsystem/1(dU/dt) -> Mux6/1, U0/1  "dU/dt"
  Subsystem1/1(dV/dt) -> Mux6/2, V0/1  "dV/dt"
  Demux2/1 -> Subsystem2/3(P), Subsystem1/3(P)
  U0/1 -> Subsystem2/5(U), Subsystem1/5(U), Mux3/1  "U"
  Demux/1 -> Subsystem/2(Fx)  "Fx"
  m/1 -> Subsystem2/1(m), Subsystem/1(m), Subsystem1/1(m)
  Demux2/2 -> Subsystem/3(Q), Subsystem2/4(Q)
  W0/1 -> Subsystem/6(W), Subsystem1/6(W), Mux3/3  "W"
  Demux/2 -> Subsystem1/2(Fy)  "Fy"
  Mux6/1 -> AAb/1
  Fxyz/1 -> Demux/1
  Mux3/1 -> Vb/1
  ωb/1 -> Demux2/1

== system quad_12_1_r2021a/Plant(UAV EOM)(Non-linear)/6DOF CORE/Subsystem6 ==
  ωb : Inport
  Demux : Demux  Outputs=3
  MATLAB Function : MATLAB Function  TreatAsAtomicUnit=on
  MATLAB Function1 : MATLAB Function  TreatAsAtomicUnit=on
  MATLAB Function2 : MATLAB Function  TreatAsAtomicUnit=on
  Mux1 : Mux  Inputs=3
  θ0 : Integrator
  φ0 : Integrator
  ψ0 : Integrator
  ΦΘΨ : Outport
  wires:
  ωb/1 -> Demux/1
  Demux/1 -> MATLAB Function/1(P)
  Demux/2 -> MATLAB Function/2(Q), MATLAB Function2/1(Q), MATLAB Function1/1(Q)
  Demux/3 -> MATLAB Function/3(R), MATLAB Function2/2(R), MATLAB Function1/2(R)
  MATLAB Function/1(phidot) -> φ0/1  "dΦ/dt"
  φ0/1 -> Mux1/1, MATLAB Function2/3(phi), MATLAB Function1/3(phi), MATLAB Function/4(phi)  "Φ"
  Mux1/1 -> ΦΘΨ/1
  θ0/1 -> Mux1/2, MATLAB Function2/4(theta), MATLAB Function/5(theta)  "Θ"
  MATLAB Function1/1(thetadot) -> θ0/1  "dΘ/dt"
  ψ0/1 -> Mux1/3  "Ψ"
  MATLAB Function2/1(pusaidot) -> ψ0/1  "dΨ/dt"

== system quad_12_1_r2021a/Plant(UAV EOM)(Non-linear)/6DOF CORE/Subsystem7 ==
  Vb : Inport
  Euler Angles : Inport  Port=2
  Mux : Mux  Inputs=3
  Subsystem : Subsystem
  Subsystem1 : Subsystem
  Subsystem2 : Subsystem
  Ve : Outport
  wires:
  Mux/1 -> Ve/1
  Euler Angles/1 -> Subsystem/2(Euler Angles), Subsystem1/2(Euler Angles), Subsystem2/2(Euler Angles)
  Vb/1 -> Subsystem/1(Vb), Subsystem2/1(Vb), Subsystem1/1(Vb)
  Subsystem/1(Vxe) -> Mux/1
  Subsystem1/1(Vye) -> Mux/2
  Subsystem2/1(Vze) -> Mux/3

== system quad_12_1_r2021a/Plant(UAV EOM)(Non-linear)/6DOF CORE/Subsystem8 ==
  Euler Angles : Inport
  MATLAB Function : MATLAB Function  TreatAsAtomicUnit=on
  DCMbe : Outport
  wires:
  MATLAB Function/1(y) -> DCMbe/1
  Euler Angles/1 -> MATLAB Function/1(u)

== system quad_12_1_r2021a/Plant(UAV EOM)(Non-linear)/6DOF CORE/Subsystem9 ==
  Ve : Inport
  Demux3 : Demux  Outputs=3
  Mux1 : Mux  Inputs=3
  Xe0 : Integrator
  Ye0 : Integrator
  Ze0 : Integrator  InitialCondition=-10
  Xe : Outport
  wires:
  Xe0/1 -> Mux1/1  "Xe"
  Ze0/1 -> Mux1/3  "Ze"
  Demux3/3 -> Ze0/1
  Demux3/2 -> Ye0/1
  Ye0/1 -> Mux1/2  "Ye"
  Demux3/1 -> Xe0/1
  Ve/1 -> Demux3/1
  Mux1/1 -> Xe/1

== system quad_12_1_r2021a/Plant(UAV EOM)(Non-linear)/6DOF CORE/Subsystem10/Subsystem ==
  m : Inport
  Fx : Inport  Port=2
  Q : Inport  Port=3
  R : Inport  Port=4
  V : Inport  Port=5
  W : Inport  Port=6
  MATLAB Function : MATLAB Function  TreatAsAtomicUnit=on
  dU/dt : Outport
  wires:
  m/1 -> MATLAB Function/1(m)
  Fx/1 -> MATLAB Function/2(Fx)
  V/1 -> MATLAB Function/3(V)
  W/1 -> MATLAB Function/4(W)
  Q/1 -> MATLAB Function/5(Q)
  R/1 -> MATLAB Function/6(R)
  MATLAB Function/1(udot) -> dU/dt/1

== system quad_12_1_r2021a/Plant(UAV EOM)(Non-linear)/6DOF CORE/Subsystem10/Subsystem1 ==
  m : Inport
  Fy : Inport  Port=2
  P : Inport  Port=3
  R : Inport  Port=4
  U : Inport  Port=5
  W : Inport  Port=6
  MATLAB Function : MATLAB Function  TreatAsAtomicUnit=on
  dV/dt : Outport
  wires:
  m/1 -> MATLAB Function/1(m)
  Fy/1 -> MATLAB Function/2(Fy)
  U/1 -> MATLAB Function/3(U)
  W/1 -> MATLAB Function/4(W)
  P/1 -> MATLAB Function/5(P)
  R/1 -> MATLAB Function/6(R)
  MATLAB Function/1(vdot) -> dV/dt/1

== system quad_12_1_r2021a/Plant(UAV EOM)(Non-linear)/6DOF CORE/Subsystem10/Subsystem2 ==
  m : Inport
  Fz : Inport  Port=2
  P : Inport  Port=3
  Q : Inport  Port=4
  U : Inport  Port=5
  V : Inport  Port=6
  MATLAB Function : MATLAB Function  TreatAsAtomicUnit=on
  dW/dt : Outport
  wires:
  m/1 -> MATLAB Function/1(m)
  Fz/1 -> MATLAB Function/2(Fz)
  U/1 -> MATLAB Function/3(U)
  V/1 -> MATLAB Function/4(V)
  P/1 -> MATLAB Function/5(P)
  Q/1 -> MATLAB Function/6(Q)
  MATLAB Function/1(wdot) -> dW/dt/1

== system quad_12_1_r2021a/Plant(UAV EOM)(Non-linear)/6DOF CORE/Subsystem7/Subsystem ==
  Vb : Inport
  Euler Angles : Inport  Port=2
  Demux : Demux  Outputs=3
  Demux1 : Demux  Outputs=3
  MATLAB Function : MATLAB Function  TreatAsAtomicUnit=on
  Vxe : Outport
  wires:
  Euler Angles/1 -> Demux1/1
  Vb/1 -> Demux/1
  Demux/1 -> MATLAB Function/1(U)
  Demux/2 -> MATLAB Function/2(V)
  Demux/3 -> MATLAB Function/3(W)
  Demux1/1 -> MATLAB Function/4(phi)
  Demux1/2 -> MATLAB Function/5(theta)
  Demux1/3 -> MATLAB Function/6(pusai)
  MATLAB Function/1(Vxe) -> Vxe/1

== system quad_12_1_r2021a/Plant(UAV EOM)(Non-linear)/6DOF CORE/Subsystem7/Subsystem1 ==
  Vb : Inport
  Euler Angles : Inport  Port=2
  Demux : Demux  Outputs=3
  Demux1 : Demux  Outputs=3
  MATLAB Function : MATLAB Function  TreatAsAtomicUnit=on
  Vye : Outport
  wires:
  Euler Angles/1 -> Demux1/1
  Vb/1 -> Demux/1
  Demux/1 -> MATLAB Function/1(U)
  Demux/2 -> MATLAB Function/2(V)
  Demux/3 -> MATLAB Function/3(W)
  Demux1/1 -> MATLAB Function/4(phi)
  Demux1/2 -> MATLAB Function/5(theta)
  Demux1/3 -> MATLAB Function/6(pusai)
  MATLAB Function/1(Vye) -> Vye/1

== system quad_12_1_r2021a/Plant(UAV EOM)(Non-linear)/6DOF CORE/Subsystem7/Subsystem2 ==
  Vb : Inport
  Euler Angles : Inport  Port=2
  Demux : Demux  Outputs=3
  Demux1 : Demux  Outputs=3
  MATLAB Function : MATLAB Function  TreatAsAtomicUnit=on
  Terminator : Terminator
  Vze : Outport
  wires:
  Euler Angles/1 -> Demux1/1
  Vb/1 -> Demux/1
  Demux/1 -> MATLAB Function/1(U)
  Demux/2 -> MATLAB Function/2(V)
  Demux/3 -> MATLAB Function/3(W)
  Demux1/1 -> MATLAB Function/4(phi)
  Demux1/2 -> MATLAB Function/5(theta)
  Demux1/3 -> Terminator/1
  MATLAB Function/1(Vze) -> Vze/1

== matlab function quad_12_1_r2021a/Plant(UAV EOM)(Non-linear)/6DOF CORE/Subsystem6/MATLAB Function ==
  data: P input; phidot output; Q input; R input; phi input; theta input
function phidot = fcn(P,Q,R,phi,theta)
    phidot = P+sin(phi)*tan(theta)*Q+cos(phi)*tan(theta)*R;
end

== matlab function quad_12_1_r2021a/Plant(UAV EOM)(Non-linear)/6DOF CORE/Subsystem6/MATLAB Function1 ==
  data: thetadot output; Q input; R input; phi input
function thetadot = fcn(Q,R,phi)
    thetadot = cos(phi)*Q-sin(phi)*R;
end

== matlab function quad_12_1_r2021a/Plant(UAV EOM)(Non-linear)/6DOF CORE/Subsystem6/MATLAB Function2 ==
  data: pusaidot output; Q input; R input; phi input; theta input
function pusaidot = fcn(Q,R,phi,theta)
    pusaidot = sin(phi)*sec(theta)*Q+cos(phi)*sec(theta)*R;
end

== matlab function quad_12_1_r2021a/Plant(UAV EOM)(Non-linear)/6DOF CORE/Subsystem7/Subsystem/MATLAB Function ==
  data: U input; Vxe output; V input; W input; phi input; theta input; pusai input
function Vxe = fcn(U,V,W,phi,theta,pusai)
    Vxe = cos(theta)*cos(pusai)*U+(sin(phi)*sin(theta)*cos(pusai)-cos(phi)*sin(pusai))*V+(cos(phi)*sin(theta)*cos(pusai)+sin(phi)*sin(pusai))*W;
end

== matlab function quad_12_1_r2021a/Plant(UAV EOM)(Non-linear)/6DOF CORE/Subsystem7/Subsystem1/MATLAB Function ==
  data: U input; Vye output; V input; W input; phi input; theta input; pusai input
function Vye = fcn(U,V,W,phi,theta,pusai)
    Vye = cos(theta)*sin(pusai)*U+(sin(phi)*sin(theta)*sin(pusai)+cos(phi)*cos(pusai))*V+(cos(phi)*sin(theta)*sin(pusai)-sin(phi)*cos(pusai))*W;
end

== matlab function quad_12_1_r2021a/Plant(UAV EOM)(Non-linear)/6DOF CORE/Subsystem7/Subsystem2/MATLAB Function ==
  data: U input; Vze output; V input; W input; phi input; theta input
function Vze = fcn(U,V,W,phi,theta)
    Vze = -sin(theta)*U+sin(phi)*cos(theta)*V+cos(phi)*cos(theta)*W;
end

== matlab function quad_12_1_r2021a/Outter Loop Controller/Position Control/MATLAB Function ==
  data: v input; vxr output; psi input; vyr output
function [vxr, vyr] = fcn(v,psi)
    vxr = cos(psi)*v(1)-sin(psi)*v(2);
    vyr = sin(psi)*v(1)+cos(psi)*v(2);
end

== matlab function quad_12_1_r2021a/Plant(UAV EOM)(Non-linear)/6DOF CORE/Subsystem8/MATLAB Function ==
  data: u input; y output
function y = fcn(u)

y = zeros(3,3);

a = u(1);
b = u(2);
c = u(3);

y(1,1) = cos(b)*cos(c);
y(1,2) = cos(b)*sin(c);
y(1,3) = -sin(b);
y(2,1) = sin(a)*sin(b)*cos(c)-cos(a)*sin(c);
y(2,2) = sin(a)*sin(b)*sin(c)+cos(a)*cos(c);
y(2,3) = sin(a)*cos(b);
y(3,1) = cos(a)*sin(b)*cos(c)+sin(a)*sin(c);
y(3,2) = cos(a)*sin(b)*sin(c)-sin(a)*cos(c);
y(3,3) = cos(a)*cos(b);

end

== matlab function quad_12_1_r2021a/Inner Loop Controller/ToRPM ==
  data: tau_x input; omega_square output; tau_y input; tau_z input; T input
function omega_square = fcn(tau_x,tau_y,tau_z,T)
    input = [tau_x;tau_y;tau_z;T];
    diameter = 0.410;
    k_tau = 1.779e-7;
    k_T = 1.097e-5;
    k = diameter/2*k_tau/sqrt(2);
    A = [-k k k -k;
        k -k k -k;
        -k_tau -k_tau k_tau k_tau;
        -k_T -k_T -k_T -k_T];
    omega_square = A\input;
end

== matlab function quad_12_1_r2021a/Plant(UAV EOM)(Non-linear)/6DOF CORE/Subsystem/MATLAB Function ==
  data: I input; P_dot output; M input size=[3,1]; omega input size=[3,1]; Q_dot output; R_dot output
function [P_dot, Q_dot, R_dot] = fcn(I,M,omega)
    omega_dot = M-cross(omega,(I*omega));
    P_dot = omega_dot(1)/I(1,1);
    Q_dot = omega_dot(2)/I(2,2);
    R_dot = omega_dot(3)/I(3,3);
end

== matlab function quad_12_1_r2021a/Actuator(Motors)1/Propeller Model ==
  data: Mb_xy output; F input; R input
function Mb_xy  = fcn(F,R)
 %%叉字型
 %3  1
 %2  4
 M_rctcm = [-sin(pi/4)*R,sin(pi/4)*R,sin(pi/4)*R,-sin(pi/4)*R;
            sin(pi/4)*R,-sin(pi/4)*R,sin(pi/4)*R,-sin(pi/4)*R];
 Mb_xy = M_rctcm*(F);%式(6.24),力矩

end

== matlab function quad_12_1_r2021a/Actuator(Motors)/Propeller Model ==
  data: Mb_xy output; F input
function Mb_xy  = fcn(F)
 %%叉字型
 %3  1
 %2  4
 R = 0.205;
 M_rctcm = [-sin(pi/4)*R,sin(pi/4)*R,sin(pi/4)*R,-sin(pi/4)*R;
            sin(pi/4)*R,-sin(pi/4)*R,sin(pi/4)*R,-sin(pi/4)*R;
            -1,-1,1,1];
 Mb_xy = M_rctcm*(F);%式(6.24),力矩

end

== matlab function quad_12_1_r2021a/Plant(UAV EOM)(Non-linear)/6DOF CORE/Subsystem10/Subsystem/MATLAB Function ==
  data: m input; udot output; Fx input; V input; W input; Q input; R input
function udot = fcn(m,Fx,V,W,Q,R)
    udot = Fx/m+R*V-Q*W;
end

== matlab function quad_12_1_r2021a/Plant(UAV EOM)(Non-linear)/6DOF CORE/Subsystem10/Subsystem1/MATLAB Function ==
  data: m input; vdot output; Fy input; U input; W input; P input; R input
function vdot = fcn(m,Fy,U,W,P,R)
    vdot = Fy/m+P*W-R*U;
end

== matlab function quad_12_1_r2021a/Plant(UAV EOM)(Non-linear)/6DOF CORE/Subsystem10/Subsystem2/MATLAB Function ==
  data: m input; wdot output; Fz input; U input; V input; P input; Q input
function wdot = fcn(m,Fz,U,V,P,Q)
    wdot = Fz/m+Q*U-P*V;
end
